simulink model "calcAeroForcesInB_th"  (R2020a)
settings: Solver=VariableStepAuto  StartTime=0.0  StopTime=timeVal(end)  RelTol=1e-3
values from neighbouring files (symbols this model uses):
  csDef = [0;0;0]*pi/180    [calcAeroCoefficients_ts.m]
  Euler = [0;180;0]*pi/180    [calcAeroCoefficients_ts.m]
  O_vWind = [0;0;0]    [calcAeroCoefficients_ts.m]
  OwB = [0;0;0]    [calcAeroCoefficients_ts.m]
libraries: calcAeroForcesInB x1, makeOcB_cl x1
settings Model: Creator=Ayaz  LastModifiedBy=Ayaz

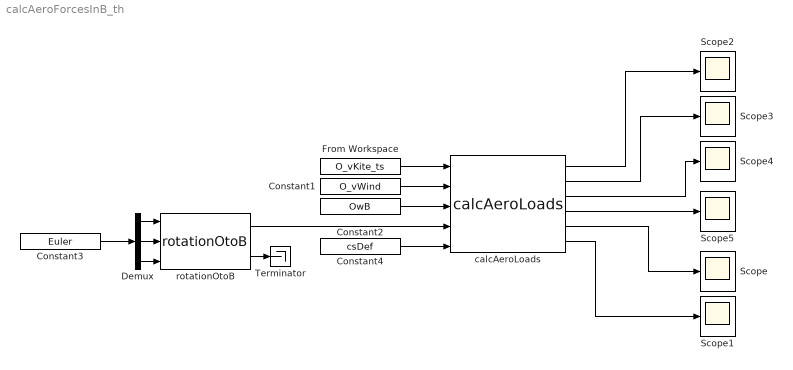
== system calcAeroForcesInB_th ==
  Constant1 : Constant  Value=O_vWind
  Constant2 : Constant  Value=OwB
  Constant3 : Constant  Value=Euler
  Constant4 : Constant  Value=csDef
  Demux : Demux  Outputs=3
  From Workspace : FromWorkspace  VariableName=O_vKite_ts
  Scope{,1..5} (6 alike) : Scope
  Terminator : Terminator
  calcAeroLoads : calcAeroForcesInB/calcAeroLoads  refChord=refChord  refSpan=refSpan  refArea=refArea  rhoAir=rhoAir
  rotationOtoB : makeOcB_cl/rotationOtoB  SystemSampleTime=-1  Latency=0  AutoFrameSizeCalculation=off
  wires:
  From Workspace/1 -> calcAeroLoads/1
  Constant1/1 -> calcAeroLoads/2
  Constant2/1 -> calcAeroLoads/3
  Constant4/1 -> calcAeroLoads/5
  calcAeroLoads/1 -> Scope2/1
  calcAeroLoads/2 -> Scope3/1
  calcAeroLoads/5 -> Scope/1
  calcAeroLoads/6 -> Scope1/1
  calcAeroLoads/3 -> Scope4/1
  calcAeroLoads/4 -> Scope5/1
  Constant3/1 -> Demux/1
  Demux/1 -> rotationOtoB/1
  Demux/2 -> rotationOtoB/2
  Demux/3 -> rotationOtoB/3
  rotationOtoB/1 -> calcAeroLoads/4
  rotationOtoB/2 -> Terminator/1
